simulink subsystem "ElectricMachine4"  (R2023a)
settings: Solver=VariableStepAuto  StartTime=0.0  StopTime=10.0  RelTol=1e-3
libraries: autolibmappedmotor x1
settings Model: ModifiedByFormat=The MathWorks, Inc.  Creator=The MathWorks, Inc.  LastModifiedBy=The MathWorks, Inc.
settings SolverCC: MaxZcPerStep=1
settings OptimizationCC: ReuseModelBlockBuffer=off
settings DebuggingCC: UnconnectedInputMsg=warning  UnconnectedOutputMsg=warning  UnconnectedLineMsg=warning
settings ModelReferenceCC: EnableRefExpFcnMdlSchedulingChecks=on
settings RTWCC: DLArmComputeVersion=19.05

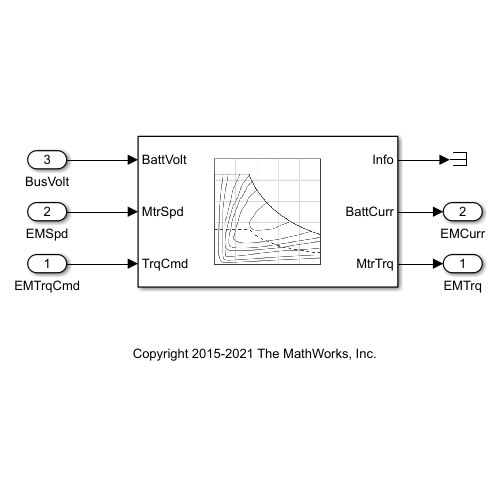
[thumbnail: Simulink's stored preview of the top-level diagram]
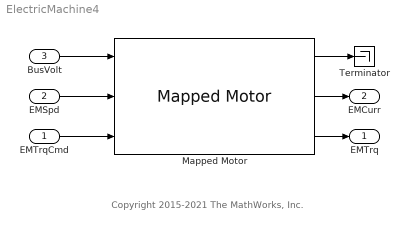
== system ElectricMachine4 ==
  note: Copyright 2015-2021 The MathWorks, Inc.
  EMTrqCmd : Inport
  EMSpd : Inport  Port=2
  BusVolt : Inport  Port=3
  Mapped Motor : autolibmappedmotor/Mapped Motor  port_config=Speed  param_by=Tabulated torque-speed envelope  w_t=PlntEM4Spd  T_t=PlntEM4Trq  torque_max=0.1  power_max=30  Tc=PlntEM4TimeCnst  param_loss=Tabulated efficiency data  eff=100  w_eff=375  T_eff=0.08  Piron=0  Pbase=0  w_eff_bp=PlntEM4Spd  T_eff_bp=PlntEM4TrqEff  Temp_eff_bp=[233.15 293.15 373.15]  losses_table=[1 2;3 4]  losses_table_3d=cat(3,1.05*[1.49 1.67 2.21 3.10; 0.42 0.69 1.14 2.03; 0.06 0.24 0.78 1.68; 0.42 0.69 1.14 2.03; 1.49 1.67 2.21 3.10],[1.49 1.67 2.21 3.10; 0.42 0.69 1.14 2.03; 0.06 0.24 0.78 1.68; 0.42 0.69 1.14 2.03; 1.49 1.67 2.21 3.10],1.03*[1.49 1.67 2.21 3.10; 0.42 0.69 1.14 2.03; 0.06 0.24 0.78 1.68; 0.42 0.69 1.14 2.03; 1.49 1.67 2.21 3.10])  efficiency_table=PlntEM4EffTbl  efficiency_table_3d=cat(3,90*ones(5,4),95*ones(5,4),92*ones(5,4))  J=5e-6  b=1e-5  omega_o=0  T_t_extended=[5.30516476972984 5.78745247606892 6.36619772367581 7.07355302630646 7.95774715459477 9.09456817667974 10.6103295394597 12.7323954473516 15.9154943091895 21.2206590789194 66.6666666666667 66.6666666666667 66.6666666666667 66.6666666666667 66.6666666666667 66.6666666666667 66.6666666666667 21.2206590789194 15.9154943091895 12.7323954473516 10.6103295394597 9.09456817667974 7.95774715459477 7.07355302630646 6.36619772367581 5.78745247606892 5.30516476972984]  w_t_extended=[-1884.95559215388 -1727.87595947439 -1570.7963267949 -1413.71669411541 -1256.63706143592 -1099.55742875643 -942.477796076938 -785.398163397448 -628.318530717959 -471.238898038469 -150 -104.71975511966 -52.3598775598299 0 52.3598775598299 104.71975511966 150 471.238898038469 628.318530717959 785.398163397448 942.477796076938 1099.55742875643 1256.63706143592 1413.71669411541 1570.7963267949 1727.87595947439 1884.95559215388]  KLossIron=0  KLossCopper=0  x_w_eff_vec=[-1884.95559215388 -1727.87595947439 -1570.7963267949 -1413.71669411541 -1256.63706143592 -1099.55742875643 -942.477796076938 -785.398163397448 -628.318530717959 -471.238898038469 -150 -104.71975511966 -52.3598775598299 0 52.3598775598299 104.71975511966 150 471.238898038469 628.318530717959 785.398163397448 942.477796076938 1099.55742875643 1256.63706143592 1413.71669411541 1570.7963267949 1727.87595947439 1884.95559215388]  x_T_eff_vec=[-66.6666666666667 -21.2206590789194 -15.9154943091895 -12.7323954473516 -10.6103295394597 -9.09456817667974 -7.95774715459477 -7.07355302630646 -6.36619772367581 -5.78745247606892 0 5.78745247606892 6.36619772367581 7.07355302630646 7.95774715459477 9.09456817667974 10.6103295394597 12.7323954473516 15.9154943091895 21.2206590789194 66.6666666666667]  x_tmp_eff_vec=[233.15 293.15 373.15]  x_losses_mat=[9458.55852693701 3010.75268817204 2258.06451612903 1806.45161290322 1505.37634408602 1290.32258064516 1129.03225806452 1003.58422939068 1186.81318681318 1775.89852008457 0 1527.27272727273 1080 933.333333333333 1050 1200 1400 1680 2099.99999999999 2800 8796.45943005142;8670.34531635892 2759.85663082437 2069.89247311827 1655.91397849462 1379.92831541219 1182.79569892473 1034.94623655914 919.95221027479 956.521739130434 1627.90697674419 0 1400 879.999999999999 855.555555555555 962.5 1100 1283.33333333333 1540 1924.99999999999 2566.66666666667 8063.4211442138;7882.13210578084 2508.9605734767 1881.72043010752 1505.37634408602 1254.48028673835 1075.2688172043 940.860215053763 836.3201911589 869.565217391303 1479.91543340381 0 1272.72727272727 799.999999999999 777.777777777777 875 1000 1166.66666666667 1400 1750 2333.33333333333 7330.38285837618;7093.91889520276 2258.06451612903 1693.54838709677 1354.83870967742 1129.03225806452 967.741935483871 846.774193548387 752.68817204301 890.109890109888 1331.92389006343 0 1145.45454545455 809.999999999999 700 787.5 900 1050 1260 1575 2100 6597.34457253856;6305.70568462467 2007.16845878136 1505.37634408602 1204.30107526881 1003.58422939068 860.215053763441 752.68817204301 669.05615292712 791.20879120879 1183.93234672304 0 1018.18181818182 719.999999999999 622.222222222222 700 800 933.333333333334 1120 1400 1866.66666666667 5864.30628670095;5517.49247404659 1756.27240143369 1317.20430107526 1053.76344086021 878.136200716846 752.68817204301 760.869565217391 676.328502415459 777.777777777777 1212.12121212121 0 1018.18181818182 699.999999999999 622.222222222222 700 700 816.666666666667 979.999999999997 1225 1633.33333333333 5131.26800086333;4729.2792634685 1505.37634408602 1129.03225806451 903.22580645161 752.688172043011 745.341614906832 741.758241758241 659.340659340658 818.181818181818 1197.33924611973 0 981.818181818181 720 600 675 685.714285714286 700 839.999999999998 1050 1400 4398.22971502571;5178.44942899416 1648.35164835165 1086.95652173913 869.565217391302 724.637681159421 706.436420722135 618.131868131868 617.283950617284 681.818181818182 997.782705099778 0 818.181818181818 600 555.555555555555 562.5 642.857142857143 666.666666666667 799.999999999998 999.999999999997 1500 4712.38898038469;5711.98664289054 1818.18181818182 1363.63636363636 888.888888888887 740.740740740742 634.920634920636 555.555555555556 606.060606060606 651.162790697674 909.090909090909 0 727.272727272727 560 533.333333333333 500 571.428571428572 666.666666666667 799.999999999998 1200 1600 5026.54824574367;5114.22059886711 1627.90697674419 1220.93023255814 818.181818181817 681.818181818183 584.415584415585 511.363636363637 454.545454545455 488.372093023256 681.818181818182 0 545.454545454545 420 400 450 514.285714285715 600.000000000001 719.999999999998 1050 1400 4398.22971502571;1904.76190476191 606.304545111983 388.63416336393 310.907330691144 217.029467852585 186.025258159358 162.772100889439 172.726294828414 155.453665345572 217.029467852584 0 173.623574282068 133.690152197192 148.544613552436 143.239448782706 163.702227180235 190.985931710275 267.380304394384 334.225380492979 509.295817894066 1600;1532.48422126331 487.804878048781 317.460317460317 253.968253968253 180.878552971576 155.038759689923 135.658914728682 120.585701981051 126.984126984127 170.940170940171 0 133.333333333333 106.666666666667 103.703703703704 116.666666666667 133.333333333333 155.555555555556 213.333333333333 266.666666666666 400 1256.63706143592;1495.99650170943 390.390390390391 263.157894736842 188.034188034188 156.695156695157 119.047619047619 91.4634146341464 81.3008130081301 83.3333333333333 85.4700854700854 0 66.6666666666666 66.6666666666666 66.6666666666666 75 95.2380952380953 122.222222222222 146.666666666666 200 288.888888888889 1047.1975511966;0 0 0 0 0 0 0 0 0 0 0 0 0 0 0 0 0 0 0 0 0;1047.1975511966 288.888888888889 200 146.666666666666 122.222222222222 95.2380952380953 75 66.6666666666666 66.6666666666666 66.6666666666666 0 ...(+3669 chars)]  x_losses_mat_3d=cat(3,[3.255 2.3205 1.7535 1.5645 1.7535 2.3205 3.255;2.1315 1.197 0.7245 0.441 0.7245 1.197 2.1315;1.764 0.819 0.252 0.063 0.252 0.819 1.764;2.1315 1.197 0.7245 0.441 0.7245 1.197 2.1315;3.255 2.3205 1.7535 1.5645 1.7535 2.3205 3.255],[3.1 2.21 1.67 1.49 1.67 2.21 3.1;2.03 1.14 0.69 0.42 0.69 1.14 2.03;1.68 0.78 0.24 0.06 0.24 0.78 1.68;2.03 1.14 0.69 0.42 0.69 1.14 2.03;3.1 2.21 1.67 1.49 1.67 2.21 3.1],[3.193 2.2763 1.7201 1.5347 1.7201 2.2763 3.193;2.0909 1.1742 0.7107 0.4326 0.7107 1.1742 2.0909;1.7304 0.8034 0.2472 0.0618 0.2472 0.8034 1.7304;2.0909 1.1742 0.7107 0.4326 0.7107 1.1742 2.0909;3.193 2.2763 1.7201 1.5347 1.7201 2.2763 3.193])  CalLossMapData={}  CalLossWithTempMapData={}  aMode=aMode  RefBlkName='autolibmappedmotor/Mapped Motor'
  Terminator : Terminator
  EMTrq : Outport  VectorParamsAs1DForOutWhenUnconnected=off
  EMCurr : Outport  Port=2  VectorParamsAs1DForOutWhenUnconnected=off
  wires:
  EMTrqCmd/1 -> Mapped Motor/3
  BusVolt/1 -> Mapped Motor/1
  EMSpd/1 -> Mapped Motor/2
  Mapped Motor/2 -> EMCurr/1
  Mapped Motor/1 -> Terminator/1
  Mapped Motor/3 -> EMTrq/1
